simulink model "SD_jf_median_control2"  (Simulink 7.3)
settings: Solver=ode1  StartTime=0.0  StopTime=Inf  FixedStep=0.001  RelTol=1e-3
PostLoadFcn:
  | , if any(exist('dsrtsu_mdlpostloadfcn', 'file') == [2, 3, 6]), try dsrtsu_mdlpostloadfcn('Execute', bdroot); catch fprintf('Error in PostLoadFcn (dsrtsu_mdlpostloadfcn) for model "%s":\n %s\n', bdroot, lasterr); end, end,
libraries: dsparch4 x6, rtilib1103 x2, simulink x2, simulink_extras x1
settings Model: DSRTSU_INTERNAL_RTI_VER=350  DSRTSU_INTERNAL_RTI_TYPE=rti1103  Creator=lewislab  LastModifiedBy=lewislab  BufferReuse=off
settings OptimizationCC: BlockReduction=off  OptimizeBlockIOStorage=off  BufferReuse=off  ExpressionFolding=off  LocalBlockOutputs=off
settings HardwareCC: ProdIntDivRoundTo=Zero  ProdEndianess=BigEndian  ProdHWDeviceType=Generic->Custom  TargetIntDivRoundTo=Zero  TargetEndianess=BigEndian  TargetHWDeviceType=Generic->Custom
settings RTWCC: SystemTargetFile=rti1103.tlc  MakeCommand=make_rti  TemplateMakefile=rti1103.tmf  Description=dSPACE DS1103 Hardware Platform  ProcessScript=rti1103_make_rtw_hook
settings STFCustomTargetCC: SystemTargetFile=rti1103.tlc
settings GRTTargetCC: ParMdlRefBuildCompliant=off  CompOptLevelCompliant=off  MatFileLogging=off  ExtModeMexFile=noextcomm
settings CustomProperty: DataType=RTWOptions_EnumType_K__Previous Projects_ForcePlate_Only_sd_jf_rti1103_1InitialSimState  Value=RUN
settings EnumStrPairs: String=RUN

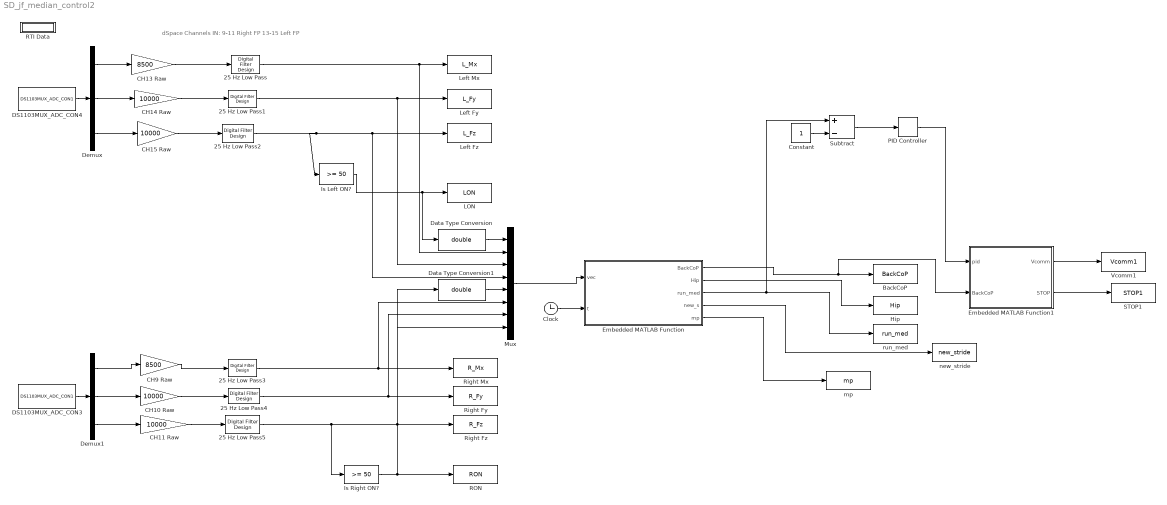
== system SD_jf_median_control2 ==
  note: dSpace Channels IN:
      | 9-11 Right FP
      | 13-15 Left FP
  25 Hz Low Pass : dsparch4/Digital Filter Design  SystemSampleTime=-1  mwdsp_browser_bugfix_var=off
      link override Digital Filter: IIRFiltStruct=Direct form II  BiQuadCoeffs=[1 2.00061135393508 1.00029855323411 1 -1.71261280567911 0.733960748872277;1 2.02501937393162 1.0253400499724 1 -1.74801194567444 0.769801128621587;1 1.99938921206706 0.999702296645625 1 -1.81742377735991 0.840078190345668;1 1.97498006006623 0.975285456788754 1 -1.91687582970982 0.94076992859855]  ScaleValues=[9.83559112410423e-010;1;1;1;1]  optimizeScaleValues=on
  25 Hz Low Pass1 : dsparch4/Digital Filter Design  SystemSampleTime=-1  mwdsp_browser_bugfix_var=off
      link override Digital Filter: IIRFiltStruct=Direct form II  BiQuadCoeffs=[1 2.00061135393508 1.00029855323411 1 -1.71261280567911 0.733960748872277;1 2.02501937393162 1.0253400499724 1 -1.74801194567444 0.769801128621587;1 1.99938921206706 0.999702296645625 1 -1.81742377735991 0.840078190345668;1 1.97498006006623 0.975285456788754 1 -1.91687582970982 0.94076992859855]  ScaleValues=[9.83559112410423e-010;1;1;1;1]  optimizeScaleValues=on
  25 Hz Low Pass2 : dsparch4/Digital Filter Design  SystemSampleTime=-1  mwdsp_browser_bugfix_var=off
      link override Digital Filter: IIRFiltStruct=Direct form II  BiQuadCoeffs=[1 2.00061135393508 1.00029855323411 1 -1.71261280567911 0.733960748872277;1 2.02501937393162 1.0253400499724 1 -1.74801194567444 0.769801128621587;1 1.99938921206706 0.999702296645625 1 -1.81742377735991 0.840078190345668;1 1.97498006006623 0.975285456788754 1 -1.91687582970982 0.94076992859855]  ScaleValues=[9.83559112410423e-010;1;1;1;1]  optimizeScaleValues=on
  25 Hz Low Pass3 : dsparch4/Digital Filter Design  SystemSampleTime=-1  mwdsp_browser_bugfix_var=off
      link override Digital Filter: IIRFiltStruct=Direct form II  BiQuadCoeffs=[1 2.00061135393508 1.00029855323411 1 -1.71261280567911 0.733960748872277;1 2.02501937393162 1.0253400499724 1 -1.74801194567444 0.769801128621587;1 1.99938921206706 0.999702296645625 1 -1.81742377735991 0.840078190345668;1 1.97498006006623 0.975285456788754 1 -1.91687582970982 0.94076992859855]  ScaleValues=[9.83559112410423e-010;1;1;1;1]  optimizeScaleValues=on
  25 Hz Low Pass4 : dsparch4/Digital Filter Design  SystemSampleTime=-1  mwdsp_browser_bugfix_var=off
      link override Digital Filter: IIRFiltStruct=Direct form II  BiQuadCoeffs=[1 2.00061135393508 1.00029855323411 1 -1.71261280567911 0.733960748872277;1 2.02501937393162 1.0253400499724 1 -1.74801194567444 0.769801128621587;1 1.99938921206706 0.999702296645625 1 -1.81742377735991 0.840078190345668;1 1.97498006006623 0.975285456788754 1 -1.91687582970982 0.94076992859855]  ScaleValues=[9.83559112410423e-010;1;1;1;1]  optimizeScaleValues=on
  25 Hz Low Pass5 : dsparch4/Digital Filter Design  SystemSampleTime=-1  mwdsp_browser_bugfix_var=off
      link override Digital Filter: IIRFiltStruct=Direct form II  BiQuadCoeffs=[1 2.00061135393508 1.00029855323411 1 -1.71261280567911 0.733960748872277;1 2.02501937393162 1.0253400499724 1 -1.74801194567444 0.769801128621587;1 1.99938921206706 0.999702296645625 1 -1.81742377735991 0.840078190345668;1 1.97498006006623 0.975285456788754 1 -1.91687582970982 0.94076992859855]  ScaleValues=[9.83559112410423e-010;1;1;1;1]  optimizeScaleValues=on
  BackCoP : ToWorkspace  VariableName=BackCoP  SampleTime=-1  SaveFormat=Array
  CH10 Raw : Gain  Gain=10000  ParameterDataType=sfix(16)  ParameterScaling=2^0  OutDataType=sfix(16)  OutScaling=2^0  SaturateOnIntegerOverflow=on  OutDataTypeStr=Inherit: Same as input  ParamDataTypeStr=Inherit: Same as input
  CH11 Raw : Gain  Gain=10000  ParameterDataType=sfix(16)  ParameterScaling=2^0  OutDataType=sfix(16)  OutScaling=2^0  SaturateOnIntegerOverflow=on  OutDataTypeStr=Inherit: Same as input  ParamDataTypeStr=Inherit: Same as input
  CH13 Raw : Gain  Gain=8500  ParameterDataType=sfix(16)  ParameterScaling=2^0  OutDataType=sfix(16)  OutScaling=2^0  SaturateOnIntegerOverflow=on  OutDataTypeStr=Inherit: Same as input  ParamDataTypeStr=Inherit: Same as input
  CH14 Raw : Gain  Gain=10000  ParameterDataType=sfix(16)  ParameterScaling=2^0  OutDataType=sfix(16)  OutScaling=2^0  SaturateOnIntegerOverflow=on  OutDataTypeStr=Inherit: Same as input  ParamDataTypeStr=Inherit: Same as input
  CH15 Raw : Gain  Gain=10000  ParameterDataType=sfix(16)  ParameterScaling=2^0  OutDataType=sfix(16)  OutScaling=2^0  SaturateOnIntegerOverflow=on  OutDataTypeStr=Inherit: Same as input  ParamDataTypeStr=Inherit: Same as input
  CH9 Raw : Gain  Gain=8500  ParameterDataType=sfix(16)  ParameterScaling=2^0  OutDataType=sfix(16)  OutScaling=2^0  SaturateOnIntegerOverflow=on  OutDataTypeStr=Inherit: Same as input  ParamDataTypeStr=Inherit: Same as input
  Clock : Clock
      settings: Decimation=10
  Constant : Constant  OutDataType=fixdt(1, 16)  OutScaling=2^0
  DS1103MUX_ADC_CON3 : rtilib1103/DS1103 MASTER PPC/DS1103MUX_ADC_CON1  SystemSampleTime=-1  ConverterNo=3  ChannelNos=[1 2 3]  TimerAPreTrigger=0  Reserved2=[]  Reserved3=[]  Reserved4=[]  DialogFcn=gui1103mux_adc  UnitName={ 'DS1103MUX_ADC_CON' }  UnitValues={ 3 }  DSProperties=struct('RTI',struct('Version',uint32(1),'BlockType',struct('isSLSource',uint8(1),'isSLSink',uint8(0),'isHWSource',uint8(1),'isHWSink',uint8(0),'isSetup',uint8(0),'isInline',uint8(1),'isNonInline',uint8(0),'isInterrupt',uint8(0),'isChannelwise',uint8(0)),'IOBoardType','DS1103MASTER','UnitType','ADC','Identifier','ADCMUX','DialogType','ML','BlockSet','NONE','SlaveProcessor','NONE'))
  DS1103MUX_ADC_CON4 : rtilib1103/DS1103 MASTER PPC/DS1103MUX_ADC_CON1  SystemSampleTime=-1  ConverterNo=4  ChannelNos=[1 2 3]  TimerAPreTrigger=0  Reserved2=[]  Reserved3=[]  Reserved4=[]  DialogFcn=gui1103mux_adc  UnitName={ 'DS1103MUX_ADC_CON' }  UnitValues={ 4 }  DSProperties=struct('RTI',struct('Version',uint32(1),'BlockType',struct('isSLSource',uint8(1),'isSLSink',uint8(0),'isHWSource',uint8(1),'isHWSink',uint8(0),'isSetup',uint8(0),'isInline',uint8(1),'isNonInline',uint8(0),'isInterrupt',uint8(0),'isChannelwise',uint8(0)),'IOBoardType','DS1103MASTER','UnitType','ADC','Identifier','ADCMUX','DialogType','ML','BlockSet','NONE','SlaveProcessor','NONE'))
  Data Type Conversion : DataTypeConversion  OutDataTypeMode=double  OutDataTypeStr=double
  Data Type Conversion1 : DataTypeConversion  OutDataTypeMode=double  OutDataTypeStr=double
  Demux : Demux  Outputs=3
  Demux1 : Demux  Outputs=3
  Embedded MATLAB Function : Stateflow chart  TreatAsAtomicUnit=on
  Embedded MATLAB Function1 : Stateflow chart  TreatAsAtomicUnit=on
  Hip : ToWorkspace  VariableName=Hip  SampleTime=-1  SaveFormat=Array
  Is Left ON? : simulink/Logic and Bit Operations/Compare To Constant  SystemSampleTime=-1  relop=>=  const=50  LogicOutDataTypeMode=uint8  ZeroCross=off
  Is Right ON? : simulink/Logic and Bit Operations/Compare To Constant  SystemSampleTime=-1  relop=>=  const=50  LogicOutDataTypeMode=uint8  ZeroCross=off
  LON : ToWorkspace  VariableName=LON  SampleTime=-1  SaveFormat=Array
  Left Fy : ToWorkspace  VariableName=L_Fy  SampleTime=-1  SaveFormat=Array
  Left Fz : ToWorkspace  VariableName=L_Fz  SampleTime=-1  SaveFormat=Array
  Left Mx : ToWorkspace  VariableName=L_Mx  SampleTime=-1  SaveFormat=Array
  Mux : Mux  Inputs=8
  PID Controller : simulink_extras/Additional Linear/PID Controller  SystemSampleTime=-1  P=3.2  I=.5  D=1.9
  RON : ToWorkspace  VariableName=RON  SampleTime=-1  SaveFormat=Array
  RTI Data : Subsystem  Tag=struct('RTIDataServer',struct('RTIDataServerVs','2','RTIModelDescription','struct(''main'',''SD_jf_median_control2'',''sub'','''',''isMp'',0)'))  LoadFcn="if exist('rtidc'), try,  rtidc('DataHostBlockClbLoad', gcbh); catch, disp(['Warning: ''LoadFcn'' for RTI Data block failed: ' lasterr]); end, end,"
      settings: CopyFcn="if exist('rtidc'), try,  rtidc('DataHostBlockClbCopy', gcbh); catch, disp(['Warning: ''CopyFcn'' for RTI Data block failed: ' lasterr]); end, end,"  DeleteFcn="if exist('rtidc'), try,  rtidc('DataHostBlockClbDelete', gcbh); catch, disp(['Warning: ''DeleteFcn'' for RTI Data block failed: ' lasterr]); end, end,"  ModelCloseFcn="if exist('rtidc'), try,  rtidc('DataHostBlockClbModelClose', gcbh); catch, disp(['Warning: ''ModelCloseFcn'' for RTI Data block failed: ' lasterr]); end, end,"  PreSaveFcn="if exist('rtidc'), try,  rtidc('DataHostBlockClbPreSave', gcbh); catch, disp(['Warning: ''PreSaveFcn'' for RTI Data block failed: ' lasterr]); end, end,"  PostSaveFcn="if exist('rtidc'), try,  rtidc('DataHostBlockClbPostSave', gcbh); catch, disp(['Warning: ''PostSaveFcn'' for RTI Data block failed: ' lasterr]); end, end,"  NameChangeFcn="if exist('rtidc'), try,  rtidc('DataHostBlockClbNameChange', gcbh); catch, disp(['Warning: ''NameChangeFcn'' for RTI Data block failed: ' lasterr]); end, end,"
      mask Type: RTI_DATA_HOST
      mask Description:
      | RTI Data Block.
      | This block is used by RTI to store internal model-dependent data.
      | Please keep this block on the root level of the model. Deleting this block will result in data loss.
      | 
      | NEVER DELETE OR COPY THIS BLOCK!
      mask Help:
      | RTI Data Block.
      | This block is used by RTI to store internal model-dependent data.
      | Please keep this block on the root level of the model. Deleting this block will result in data loss.
      | 
      | NEVER DELETE OR COPY THIS BLOCK!
      mask Display:
      | text(0.5, 0.5, 'RTI Data', 'HorizontalAlignment', 'center');
      | plot([1 0]);
  Right Fy : ToWorkspace  VariableName=R_Fy  SampleTime=-1  SaveFormat=Array
  Right Fz : ToWorkspace  VariableName=R_Fz  SampleTime=-1  SaveFormat=Array
  Right Mx : ToWorkspace  VariableName=R_Mx  SampleTime=-1  SaveFormat=Array
  STOP1 : ToWorkspace  VariableName=STOP1  SampleTime=-1  SaveFormat=Array
  Subtract : Sum  Inputs=+-  OutDataType=fixdt(1, 16)  OutScaling=2^-10
  Vcomm1 : ToWorkspace  VariableName=Vcomm1  SampleTime=-1  SaveFormat=Array
  mp : ToWorkspace  VariableName=mp  SampleTime=-1  SaveFormat=Array
  new_stride : ToWorkspace  VariableName=new_stride  SampleTime=-1  SaveFormat=Array
  run_med : ToWorkspace  VariableName=run_med  SampleTime=-1  SaveFormat=Array
  wires:
  Is Left ON?/1 -> LON/1, Data Type Conversion/1
  Is Right ON?/1 -> RON/1, Data Type Conversion1/1
  Mux/1 -> Embedded MATLAB Function/1(vec)
  Data Type Conversion/1 -> Mux/1
  Data Type Conversion1/1 -> Mux/5
  Embedded MATLAB Function/1(BackCoP) -> Embedded MATLAB Function1/2(BackCoP), BackCoP/1
  Embedded MATLAB Function/2(Hip) -> Hip/1
  25 Hz Low Pass/1 -> Mux/2, Left Mx/1
  25 Hz Low Pass1/1 -> Mux/3, Left Fy/1
  25 Hz Low Pass2/1 -> Is Left ON?/1, Mux/4, Left Fz/1
  25 Hz Low Pass3/1 -> Mux/6, Right Mx/1
  25 Hz Low Pass4/1 -> Mux/7, Right Fy/1
  25 Hz Low Pass5/1 -> Is Right ON?/1, Mux/8, Right Fz/1
  Clock/1 -> Embedded MATLAB Function/2(t)
  Embedded MATLAB Function/3(run_med) -> Subtract/1, run_med/1
  DS1103MUX_ADC_CON4/1 -> Demux/1
  Demux/1 -> CH13 Raw/1
  Demux/2 -> CH14 Raw/1
  DS1103MUX_ADC_CON3/1 -> Demux1/1
  Demux/3 -> CH15 Raw/1
  CH14 Raw/1 -> 25 Hz Low Pass1/1
  CH15 Raw/1 -> 25 Hz Low Pass2/1
  Demux1/1 -> CH9 Raw/1
  Demux1/2 -> CH10 Raw/1
  Demux1/3 -> CH11 Raw/1
  CH9 Raw/1 -> 25 Hz Low Pass3/1
  CH10 Raw/1 -> 25 Hz Low Pass4/1
  CH11 Raw/1 -> 25 Hz Low Pass5/1
  Embedded MATLAB Function/4(new_s) -> new_stride/1
  Embedded MATLAB Function/5(mp) -> mp/1
  Embedded MATLAB Function1/1(Vcomm) -> Vcomm1/1
  Embedded MATLAB Function1/2(STOP) -> STOP1/1
  PID Controller/1 -> Embedded MATLAB Function1/1(pid)
  Subtract/1 -> PID Controller/1
  CH13 Raw/1 -> 25 Hz Low Pass/1
  Constant/1 -> Subtract/2

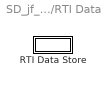
== system SD_jf_median_control2/RTI Data ==
  RTI Data Store : Subsystem  Tag="struct('public',struct('sub',struct('name',{{'SD_jf_median_control2'}},'data',{{struct('TH',struct('thTaskInfo',struct('taskType',{'TIMER','HWINT','TMRINT','SWINT'},'tasksNumOf',{1,0,0,0},'srcIds',{{'TIMERA'},{},{},{}},'taskNames',{{['Timer Task 1']},{},{},{}})),'th_tc',struct('dataType','TASK','taskGroupId','','taskGroupList',{{}},'taskSchedulingPolicy','FCFS','taskType','TIMER','blkh',-1,'srcId','TIMERA','srcSgnName',['Timer A interrupt'],'srcCpuName','','taskName',['Timer Task 1  [0.001] s'],'taskNameDisplayExt','','smplTime',0.001,'smplTimeOffs',0,'hasFixedPriority',0,'priority',1,'hasFixedOvc',0,'ovcType',1,'ovcMax',1),'tc_th',struct('dataType','TASK','taskGroupId','','taskGroupList',{{}},'taskSchedulingPolicy','FCFS','taskType','TIMER','blkh',-1,'srcId','TIMERA','srcSgnName',['Timer A interrupt'],'srcCpuName','','taskName',['Timer Task 1  [0.001] s'],'taskNameDisplayExt','','smplTime',0.001,'smplTimeOffs',0,'hasFixedPriority',0,'priority',1,'hasFixedOvc',0,'ovcType',1,'ovcMax',1))}})),'private',struct('version',struct('dsVer',uint32(2)),'access',struct('modified',['12-Apr-2017 15:52:02'],'type','Model','isPerm',1)))"
      mask Type: RTI_DATA_STORE
      mask Description:
      | RTI Data Store Block. This block is used by RTI to store internal model dependent data. Deleting this block will result in data loss.
      | 
      | NEVER DELETE, COPY, OR MODIFY THIS BLOCK!
      mask Help:
      | RTI Data Store Block. This block is used by RTI to store internal model dependent data. Deleting this block will result in data loss.
      | 
      | NEVER DELETE, COPY, OR MODIFY THIS BLOCK!
      mask Display: text(0.5, 0.5, ' ', 'HorizontalAlignment', 'center');

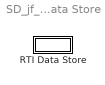
== system SD_jf_median_control2/RTI Data/RTI Data Store ==
  RTI Data Store : Subsystem
      mask Type: RTI_DATA_STORE
      mask Description:
      | RTI Data Store Block. This block is used by RTI to store internal model dependent data. Deleting this block will result in data loss.
      | 
      | NEVER DELETE, COPY, OR MODIFY THIS BLOCK!
      mask Help:
      | RTI Data Store Block. This block is used by RTI to store internal model dependent data. Deleting this block will result in data loss.
      | 
      | NEVER DELETE, COPY, OR MODIFY THIS BLOCK!
      mask Display: text(0.5, 0.5, ' ', 'HorizontalAlignment', 'center');

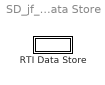
== system SD_jf_median_control2/RTI Data/RTI Data Store/RTI Data Store ==
  RTI Data Store : Subsystem
      mask Type: RTI_DATA_STORE
      mask Description:
      | RTI Data Store Block. This block is used by RTI to store internal model dependent data. Deleting this block will result in data loss.
      | 
      | NEVER DELETE, COPY, OR MODIFY THIS BLOCK!
      mask Help:
      | RTI Data Store Block. This block is used by RTI to store internal model dependent data. Deleting this block will result in data loss.
      | 
      | NEVER DELETE, COPY, OR MODIFY THIS BLOCK!
      mask Display: text(0.5, 0.5, ' ', 'HorizontalAlignment', 'center');

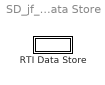
== system SD_jf_median_control2/RTI Data/RTI Data Store/RTI Data Store/RTI Data Store ==
  RTI Data Store : Subsystem
      mask Type: RTI_DATA_STORE
      mask Description:
      | RTI Data Store Block. This block is used by RTI to store internal model dependent data. Deleting this block will result in data loss.
      | 
      | NEVER DELETE, COPY, OR MODIFY THIS BLOCK!
      mask Help:
      | RTI Data Store Block. This block is used by RTI to store internal model dependent data. Deleting this block will result in data loss.
      | 
      | NEVER DELETE, COPY, OR MODIFY THIS BLOCK!
      mask Display: text(0.5, 0.5, ' ', 'HorizontalAlignment', 'center');

== system SD_jf_median_control2/RTI Data/RTI Data Store/RTI Data Store/RTI Data Store/RTI Data Store ==

== matlab function Embedded MATLAB Function1 ==
  data: pid input double; BackCoP input double; Vcomm output double; STOP output double

function [Vcomm, STOP]  = safety(pid,BackCoP)
    %dt = .001;
    persistent thrown
    persistent curr_speed
    
     if isempty(curr_speed)
         curr_speed = 0;
     end
%         
    if isempty(thrown)
        thrown = 0;
    end
    
    if (thrown == 1)
        Vadd = 0;
        curr_speed = 0;
    
    elseif (BackCoP <= 0.3) %safety condition
        thrown = 1;
        Vadd = 0;
        curr_speed = 0;
        
    else %normal function as PID controller of belt speed
        if abs(pid - curr_speed) <= .002
            Vadd = pid;
        else
            Vadd = curr_speed + .002 * sign(pid - curr_speed);
        end
    end
    
    STOP = thrown;
    %Vcomm = curr_speed + (Vadd * dt);    
    Vcomm = Vadd; %*dt
    curr_speed = Vcomm;
    
end

== matlab function Embedded MATLAB Function ==
  data: vec input double; BackCoP output double; Hip output double; run_med output double; t input double; new_s output double; mp output double
    function [BackCoP, Hip, run_med, new_s, mp] = data_parse4(vec,t)
        offset = .02295; %Right plate offset from origin
        BackCoP = 1;
        Hip = 1;
        L = .85; %leg length
        persistent I
        if isempty(I)
            I=0;
        end
        persistent new_stride
        if isempty(new_stride)
           new_stride = 0; 
        end
        y0 = 1;
        rf = 600;
        persistent curr_struct
        if isempty(curr_struct)
            curr_struct = struct('slide', y0*ones(rf,1),'run_med',y0,...
            'last_state',1,'maxFz',200,'mp_vec',y0*ones(3,1),'stride',y0,...
            'len',0,'stime', zeros(3,1)); 
        end

          %manually demux the collected signals
        LON = vec(1);
        LMx = vec(2);
        LFy = vec(3);
        LFz = vec(4);
        RON = vec(5);
        RMx = vec(6);
        RFy = vec(7);
        RFz = vec(8);

        persistent minFz
        if isempty(minFz)
            minFz = 600;
        end


        if (LON==1 && RON ==1) %double support
            minFz = 600;
            LCoP = LMx / LFz;
            RCoP = (RMx / RFz) + offset;
            if (RCoP < LCoP) % Right is back leg
                BackCoP = RCoP;
                Hip = BackCoP - L*(RFy / sqrt(RFy^2 + max(RFz,minFz)^2));

                BackFz = RFz;
            else % Left is back leg
                BackCoP = LCoP;
                Hip = BackCoP - (L*LFy / sqrt(LFy^2 + max(LFz,minFz)^2));

                BackFz = LFz;
            end

            %grow current stride
            curr_struct.last_state = 2;
            curr_struct.stride(curr_struct.len + 1) = Hip;
            curr_struct.len = curr_struct.len + 1;

            %sliding median
            curr_struct.slide = circshift(curr_struct.slide,1);
            curr_struct.slide(rf) = Hip;
            curr_struct.run_med = median(curr_struct.slide);
            new_stride = 0;
            if BackFz > curr_struct.maxFz
                curr_struct.maxFz = BackFz; 
            end

        elseif LON==1 % Left single support
            BackCoP = LMx / LFz;
            Hip = BackCoP - L*(LFy / sqrt(LFy^2 + max(LFz,minFz)^2));
            BackFz = LFz;

            if curr_struct.last_state == 2 %new stride detected
                %update mp_vec
                curr_struct.mp_vec = circshift(curr_struct.mp_vec',1)';
                curr_struct.mp_vec(3) = curr_struct.stride(ceil(curr_struct.len / 2));

                %rest stride
                curr_struct.stride = Hip; %holds hip data for the current stride
                curr_struct.len = 1;
                curr_struct.maxFz = BackFz;
                curr_struct.stime = circshift(curr_struct.stime',1)';
                curr_struct.stime(3) = t;
                dt = curr_struct.stime(3) - curr_struct.stime(2);
                I = I + dt * (curr_struct.mp_vec(3) - y0);

                %sliding median
                curr_struct.slide = circshift(curr_struct.slide,1);
                curr_struct.slide(rf) = Hip;
                curr_struct.run_med = median(curr_struct.slide);
                curr_struct.maxFz = BackFz;
                new_stride = 1;
            else
                %grow current stride
                curr_struct.stride(curr_struct.len + 1) = Hip;
                curr_struct.len = curr_struct.len + 1;

                %sliding median
                curr_struct.slide = circshift(curr_struct.slide,1);
                curr_struct.slide(rf) = Hip;
                curr_struct.run_med = median(curr_struct.slide);
                curr_struct.maxFz = BackFz;
                new_stride = 0;
                if BackFz > curr_struct.maxFz
                   curr_struct.maxFz = BackFz; 
                end
            end

            curr_struct.last_state = 1;
        elseif (RON == 1) % Right Single support
            BackCoP = (RMx / RFz) + offset;
            Hip = BackCoP - L*(RFy / sqrt(RFy^2 + max(RFz,minFz)^2));

            BackFz = RFz;

            if curr_struct.last_state == 2 %new stride detected
                %update mp_vec
                curr_struct.mp_vec = circshift(curr_struct.mp_vec',1)';
                curr_struct.mp_vec(3) = curr_struct.stride(ceil(curr_struct.len / 2));

                %reset stride
                curr_struct.stride = Hip; %holds hip data for the current stride
                curr_struct.len = 1;
                curr_struct.maxFz = BackFz;
                curr_struct.stime = circshift(curr_struct.stime',1)';
                curr_struct.stime(3) = t;

                dt = curr_struct.stime(3) - curr_struct.stime(2);
                I = I + dt * (curr_struct.mp_vec(3) - y0);

                %sliding median
                curr_struct.slide = circshift(curr_struct.slide,1);
                curr_struct.slide(rf) = Hip;
                curr_struct.run_med = median(curr_struct.slide);
                curr_struct.maxFz = BackFz;
                new_stride = 1;
            else
                %grow current stride
                curr_struct.stride(curr_struct.len + 1) = Hip;
                curr_struct.len = curr_struct.len + 1;

                %sliding median
                curr_struct.slide = circshift(curr_struct.slide,1);
                curr_struct.slide(rf) = Hip;
                curr_struct.run_med = median(curr_struct.slide);
                curr_struct.maxFz = BackFz;
                new_stride = 0;
                if BackFz > curr_struct.maxFz
                   curr_struct.maxFz = BackFz; 
                end
            end

            curr_struct.last_state = 1;
        else % float
            %reset stride
             minFz = 600;
             curr_struct.stride = Hip; %holds hip data for the current stride
             curr_struct.len = 1;
             curr_struct.stime = circshift(curr_struct.stime',1)';
             curr_struct.stime(3) = t;

             dt = curr_struct.stime(3) - curr_struct.stime(2);
             I = I + dt * (curr_struct.mp_vec(3) - y0);

             %sliding median (set based on assuming person stays at median of last stride)
             curr_struct.slide = circshift(curr_struct.slide,1);
             curr_struct.slide(rf) = curr_struct.mp_vec(3);
             %curr_struct.run_med = curr_struct.mp_vec(3);

             curr_struct.run_med  =  curr_struct.run_med;
             curr_struct.slide = circshift(curr_struct.slide,1);
             curr_struct.slide(rf) = curr_struct.run_med;

             new_stride = 1;
             curr_struct.last_state = 2;
        end
        minFz = .8 * curr_struct.maxFz;
      %manual  triggered PID    
        V = diff(curr_struct.mp_vec) ./ diff(curr_struct.stime); %velocity of last two strides
        Pcurr = curr_struct.mp_vec(3) - y0; %most recent position error
        Icurr = I; %integral error
        Dcurr = V(2);% most recent velocity  (of error)

        mp = curr_struct.mp_vec(3);
        run_med = curr_struct.run_med;
        new_s = new_stride;
    end
